simulink model "ch_5_7_dsb"  (Simulink 6.3)
settings: Solver=ode45  StartTime=0.0  StopTime=10  RelTol=1e-3
values from neighbouring files (symbols this model uses):
  Fs = tf(beta,1)    [ex_16_3.m]
undefined symbols (not defined in the file or in its folder): get
libraries: dspsnks4 x3, commanapbnd3 x2
settings Model: LastModifiedBy=Yuantao Gu

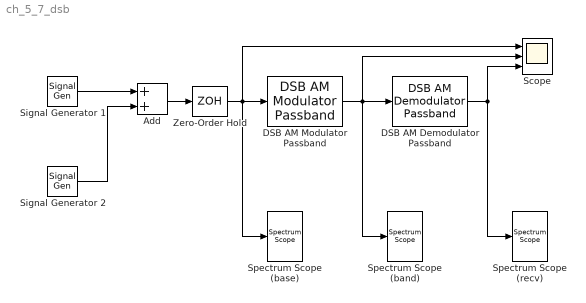
== system ch_5_7_dsb ==
  Add : Sum  OutScaling=2^-10
  DSB AM Demodulator Passband : commanapbnd3/DSB AM Demodulator Passband  Fc=100  Ph=0  method=Butterworth  n=4  cf=30  Rp=1  Rs=1  Offset=0
  DSB AM Modulator Passband : commanapbnd3/DSB AM Modulator Passband  Fc=100  Ph=0  Offset=0
  Scope : Scope  NumInputPorts=3
      settings: AttributesFormatString='r'=%<ForegroundColor>  TimeRange=1  YMin=-5~-5~-5  YMax=5~5~5
  Signal Generator 1 : SignalGenerator  Amplitude=3  Frequency=10
  Signal Generator 2 : SignalGenerator  Amplitude=2  Frequency=20
  Spectrum Scope (band) : dspsnks4/Spectrum Scope  DialogController=dspdialog.SpectrumScope  DialogControllerArgs=DataTag0  ScopeProperties=on  Domain=Frequency  HorizSpan=1  UseBuffer=on  BufferSize=512  Overlap=256  inpFftLenInherit=on  FFTlength=1024  numAvg=4  DisplayProperties=off  AxisGrid=on  Memory=off  FrameNumber=on  AxisLegend=off  AxisZoom=off  OpenScopeAtSimStart=on  OpenScopeImmediately=off  FigPos=get(0,'defaultfigureposition')  AxisProperties=off  XUnits=Hertz  XRange=[-Fs/2...Fs/2]  InheritXIncr=off  XIncr=0.002  XLabel=Samples  YUnits=Magnitude-squared  YLabel=Magnitude-squared  LineProperties=off  wintypeSpecScope=Hann  RsSpecScope=50  betaSpecScope=5  winsampSpecScope=Periodic
      settings: YMin=7.51499767475989e-012  YMax=201.190761959386
  Spectrum Scope (base) : dspsnks4/Spectrum Scope  DialogController=dspdialog.SpectrumScope  DialogControllerArgs=DataTag1  ScopeProperties=on  Domain=Frequency  HorizSpan=1  UseBuffer=on  BufferSize=512  Overlap=256  inpFftLenInherit=on  FFTlength=1024  numAvg=4  DisplayProperties=off  AxisGrid=on  Memory=off  FrameNumber=on  AxisLegend=off  AxisZoom=off  OpenScopeAtSimStart=on  OpenScopeImmediately=off  FigPos=get(0,'defaultfigureposition')  AxisProperties=off  XUnits=Hertz  XRange=[-Fs/2...Fs/2]  InheritXIncr=off  XIncr=0.002  XLabel=Samples  YUnits=Magnitude-squared  YLabel=Magnitude-squared  LineProperties=off  wintypeSpecScope=Hann  RsSpecScope=50  betaSpecScope=5  winsampSpecScope=Periodic
      settings: YMin=1.72320926221641e-014  YMax=786.250393129492
  Spectrum Scope (recv) : dspsnks4/Spectrum Scope  DialogController=dspdialog.SpectrumScope  DialogControllerArgs=DataTag2  ScopeProperties=on  Domain=Frequency  HorizSpan=1  UseBuffer=on  BufferSize=512  Overlap=256  inpFftLenInherit=on  FFTlength=1024  numAvg=4  DisplayProperties=off  AxisGrid=on  Memory=off  FrameNumber=on  AxisLegend=off  AxisZoom=off  OpenScopeAtSimStart=on  OpenScopeImmediately=off  FigPos=get(0,'defaultfigureposition')  AxisProperties=off  XUnits=Hertz  XRange=[-Fs/2...Fs/2]  InheritXIncr=off  XIncr=0.002  XLabel=Samples  YUnits=Magnitude-squared  YLabel=Magnitude-squared  LineProperties=off  wintypeSpecScope=Hann  RsSpecScope=50  betaSpecScope=5  winsampSpecScope=Periodic
      settings: YMin=1.23382686060591e-012  YMax=796.08290314563
  Zero-Order Hold : ZeroOrderHold  SampleTime=0.002
  wires:
  Signal Generator 1/1 -> Add/1
  DSB AM Modulator Passband/1 -> Spectrum Scope (band)/1, DSB AM Demodulator Passband/1, Scope/2
  DSB AM Demodulator Passband/1 -> Spectrum Scope (recv)/1, Scope/3
  Add/1 -> Zero-Order Hold/1
  Signal Generator 2/1 -> Add/2
  Zero-Order Hold/1 -> Spectrum Scope (base)/1, DSB AM Modulator Passband/1, Scope/1
